simulink model "DrivingTestBench"  (R2026a)
settings: Solver=ode3  StartTime=0  StopTime=30  FixedStep=Ts  MaxStep=Ts
PreLoadFcn:
  | if(~configureDrivingTestBench.isdrivingApplicationOnPath())
  |     pathToDrivingApplication = fullfile(...
  |         matlabshared.supportpkg.getSupportPackageRoot,...
  |         "toolbox", "driving", "supportpackages", "variantgenerator", "drivingApplication");
  | 
  | 
  |     if (~exist("pathToDrivingApplication", "dir"))
  |         sldiagviewer.reportError(['This model requires you to download and install '...
  |             'Automated Driving Toolbox™ Test Suite for Euro NCAP® Protocols']);
  |     else
  |         addpath(fullfile(matlabshared.supportpkg.getSupportPackageRoot,"toolbox", "driving", "supportpackages", "variantgenerator", "drivingApplication"));
  |     end
  | end
values from neighbouring files (symbols this model uses):
  actorProfiles = repmat(actorProfile, 1, numActors)    [configureDrivingTestBench.m]
  BusActorPoses = Simulink.Bus    [configureDrivingTestBench.m]
  egoVehDyn = egoVehicleDynamicsParams(obj, egoInitialPose, actorProfiles(egoIndex))    [configureDrivingTestBench.m]
  m = worldActors(idx).actor_runtime.pose.matrix    [configureDrivingTestBench.m]
  maxAcc = 6    [configureDrivingTestBench.m]
  n = length(i)    [TargetBehavior.m]
  testStartPosition = [egoStartXPos egoStartYPos egoStartZPos]    [configureDrivingTestBench.m]
undefined symbols (not defined in the file or in its folder): aebEnable, cameraParams, Defined, driving, dtleThreshold, Ego, egoActorID, egoPathWidth, Lane, Left, lkaEnable, matlabshared, maxDecel, maxNumActors, Right, steadyStateSpeed, trackingParams, trackPosSelector, Ts, User
libraries: roadrunnerscenario x6, simulink_extras x6, drivingscenarioandsensors x4, trackingutilitieslib x1, drivinglib x1, simulink x1, autolibutils x1, autolibshared x1
(part 2 of 2)

== matlab function DrivingTestBench/Scenario and Environment/Extract Ego Pose/Pack Ego Actor ==
  data: pos input; a output Bus: BusActorRuntime size=1; vel input; yaw input; yawRate input; egoActorID parameter
function a = packEgo(pos,vel,yaw,yawRate, egoActorID)
% Pack ego information into a single ego actor bus
%

% Initialize output struct
a = struct('ActorID', uint64(0), ...
    'Pose', zeros(4,4), ...
    'Velocity', zeros(1,3), ...
    'AngularVelocity', zeros(1,3));  % deg/sec

vehPos = [pos(1) pos(2) pos(3)]; 

Velocity = [vel(1) vel(2) 0];
AngularVelocity = [0 0 deg2rad(yawRate)];

% Get Roatational matrix
rotation = [deg2rad(yaw-90) 0 0];  % [yaw, pitch,roll] in rad
rotm = robotics.internal.eul2rotm(rotation,'ZYX'); % Convert Euler angles to rotation matrix

% Construct BusActorRuntime object
a.ActorID = uint64(egoActorID);
a.Pose(:,:) = [[rotm vehPos']; [0 0 0 1]];
a.Velocity = Velocity;     % m/s
a.AngularVelocity = AngularVelocity;  % deg/sec

== matlab function DrivingTestBench/Scenario and Environment/Extract Ego Pose/MATLAB Function1 ==
  data: u input; y output
function y = fcn(u)

y = wrapTo2Pi(u);

== matlab function DrivingTestBench/Scenario and Environment/Test Enable/Find MIO In Parallel Lanes ==
  data: confirmedTracks input; x output; positionSelector input; laneWidth input; egoPose input; vx output; mioTrack output
function [x, vx, mioTrack] = findParallelLaneMIO(confirmedTracks, positionSelector, laneWidth, egoPose)
    
    % Initialize outputs and parameters
    numStates = 6;
    maxX = cast(1000, 'like', confirmedTracks.Tracks(1).State);
    trackID = 0;
    collisionThresholdTime = 1.5;

    % Extract ego vehicle parameters
    egoVelocity = egoPose.Velocity;
   
    % Determine if the ego vehicle is attempting a lane change
    laneChangeThreshold = 0.1;
    isLaneChanging = abs(egoVelocity(2)) > laneChangeThreshold;

    if ~isLaneChanging
        x = inf;
        vx = inf;
        mioTrack = -1;
        return;
    end


    for i = 1:confirmedTracks.NumTracks
        position = positionSelector * confirmedTracks.Tracks(i).State;
        x = position(1);
        y = position(2);

        % Check if the current track is the MIO
        if x < maxX && x > 0
            yLeftParallelLane  = polyval([0, 0, 1.5 * laneWidth], x);
            yRightParallelLane = polyval([0, 0, 0.5 * laneWidth], x);

            if (yRightParallelLane <= y) && (y <= yLeftParallelLane)
                targetVelocity = confirmedTracks.Tracks(i).State(2:3);
                relativeVelocity = targetVelocity - egoVelocity(1:2);
                relativeSpeed = norm(relativeVelocity);

                if relativeSpeed > 0
                    ttc = x / relativeSpeed;
                else
                    ttc = inf;
                end

                if ttc < collisionThresholdTime
                    maxX = x;
                    trackID = i;
                end
            end
        end

    end

    % Highlight the MIO if found
    if trackID > 0
        mioState = confirmedTracks.Tracks(trackID).State;
    else
        mioState = zeros(numStates, 1, 'like', confirmedTracks.Tracks(1).State);
        mioState(1) = 500;
        mioState(2) = 0.01;
    end

    % Output:
    x = mioState(1);
    vx = mioState(2);
    mioTrack = trackID;
end

== matlab function DrivingTestBench/Scenario and Environment/Calculate TTC ==
  data: actors input; ttc output; actorProfiles parameter
function ttc =  calculateTTC(actors, actorProfiles)

% Check the number of actors
if numel(actors.Actors) == 1
    ttc = inf; % No collision possible with only one actor
    return;
end

x1 = actors.Actors.Position;
x2 = [0,0,0];
v1 = actors.Actors.Velocity;
v2 = [0,0,0];
dimension1 = [actorProfiles(1).Length,actorProfiles(1).Width, actorProfiles(1).Height];
dimension2 = [actorProfiles(2).Length,actorProfiles(2).Width, actorProfiles(2).Height];
ttc = estimateTTC(x1, v1,dimension1, x2, v2,dimension2);
end

function ttc = estimateTTC(position_1, velocity_1, dimension_1, position_2, velocity_2, dimension_2)
% Calculate the relative velocity
relativeVelocity = velocity_2 - velocity_1;

% Calculate the effective distance considering the dimensions of the vehicles
effectiveDistance = calculateEffectiveDistance(position_1, dimension_1, position_2, dimension_2);

% Ensure the effective distance is not negative
if effectiveDistance < 0
    effectiveDistance = 0;
end

% Calculate the relative speed
relativeSpeed = norm(relativeVelocity);

% Calculate TTC
ttc = effectiveDistance / relativeSpeed;

end

function effectiveDistance = calculateEffectiveDistance(position_1, dimension_1, position_2, dimension_2)
% Calculate the half dimensions
halfDim1 = dimension_1 / 2;
halfDim2 = dimension_2 / 2;

% Calculate the min and max coordinates for each vehicle
minCoords1 = position_1 - halfDim1;
maxCoords1 = position_1 + halfDim1;
minCoords2 = position_2 - halfDim2;
maxCoords2 = position_2 + halfDim2;

% Calculate the overlap in each dimension
overlapX = max(0, min(maxCoords1(1), maxCoords2(1)) - max(minCoords1(1), minCoords2(1)));
overlapY = max(0, min(maxCoords1(2), maxCoords2(2)) - max(minCoords1(2), minCoords2(2)));
overlapZ = max(0, min(maxCoords1(3), maxCoords2(3)) - max(minCoords1(3), minCoords2(3)));

% Calculate the effective distance
effectiveDistanceX = max(0, abs(position_2(1) - position_1(1)) - (halfDim1(1) + halfDim2(1) - overlapX));
effectiveDistanceY = max(0, abs(position_2(2) - position_1(2)) - (halfDim1(2) + halfDim2(2) - overlapY));
effectiveDistanceZ = max(0, abs(position_2(3) - position_1(3)) - (halfDim1(3) + halfDim2(3) - overlapZ));

% Combine the effective distances
effectiveDistance = norm([effectiveDistanceX, effectiveDistanceY, effectiveDistanceZ]);
end

== matlab function DrivingTestBench/Scenario and Environment/Extract Ego Pose/Center To Rear Axle ==
  data: actorRuntime input; actorPose output Bus: BusActorPose; CGToRearAxle parameter
function actorPose = centerToRearAxle(actorRuntime,CGToRearAxle)
% centerToRearAxle function converts BusActorRuntime format to driving
% scenario compatable format.

% Initialize output struct
actorPose = struct('ActorID', 0, ...
    'Position', zeros([1,3]), ...
    'Velocity', zeros([1,3]), ...
    'Roll', 0, ...  % deg
    'Pitch', 0, ... % deg
    'Yaw', 0, ...   % deg
    'AngularVelocity', zeros([1,3]));  % deg/sec

% Get pose from rotation matrix
rotationMatrix = actorRuntime.Pose(1:3,1:3);
rotation = robotics.internal.rotm2eul(rotationMatrix,'ZYX'); % The default order for Euler angle rotations is "ZYX"
rotation = rad2deg(rotation);
vehPos = actorRuntime.Pose(1:3,4)';

yaw = rotation(1) + 90;

% Translate position from center of the vehicle to one
% located under the rear axle.
% yaw must be in degrees.

forwardVector = [cosd(yaw) sind(yaw) 0];
newPos = vehPos - CGToRearAxle*forwardVector;

% Construct output struct
actorPose.ActorID  = double(actorRuntime.ActorID);
actorPose.Position = newPos;
actorPose.Velocity = actorRuntime.Velocity;
actorPose.Roll     = rotation(3);
actorPose.Pitch    = rotation(2);
actorPose.Yaw      = yaw;
actorPose.AngularVelocity = rad2deg(actorRuntime.AngularVelocity);
